simulink model "three_time_scale"  (R2015a)
settings: Solver=ode45  StartTime=0.0  StopTime=30000.0  RelTol=1e-3
values from neighbouring files (symbols this model uses):
  alpha = 0.25    [fast_nullcline_winged_cusp.m]    (also in relay_model_bistability.m; relay_model_bistability2.m)
  beta = 0.5    [fast_nullcline_winged_cusp.m]    (also in relay_model_bistability.m; relay_model_bistability2.m = 0.25)
  delta = 0.5    [fast_nullcline_winged_cusp.m]    (also in relay_model_bistability.m = 0.3; relay_model_bistability2.m = 0.3)
  gamma = 0.5    [fast_nullcline_winged_cusp.m]    (also in relay_model_bistability.m = 1; relay_model_bistability2.m = 1)
undefined symbols (not defined in the file or in its folder): xu
libraries: simulink x1
settings Model: CovModelRefEnable=off  Creator=rajiv  LastModifiedBy=rajiv
settings DataIOCC: SaveFormat=Dataset
settings HardwareCC: ProdBitPerPointer=64  ProdLargestAtomicFloat=Float  ProdIntDivRoundTo=Zero  ProdEndianess=LittleEndian  ProdHWDeviceType=Specified
settings GRTTargetCC: GeneratePreprocessorConditionals=Use local settings

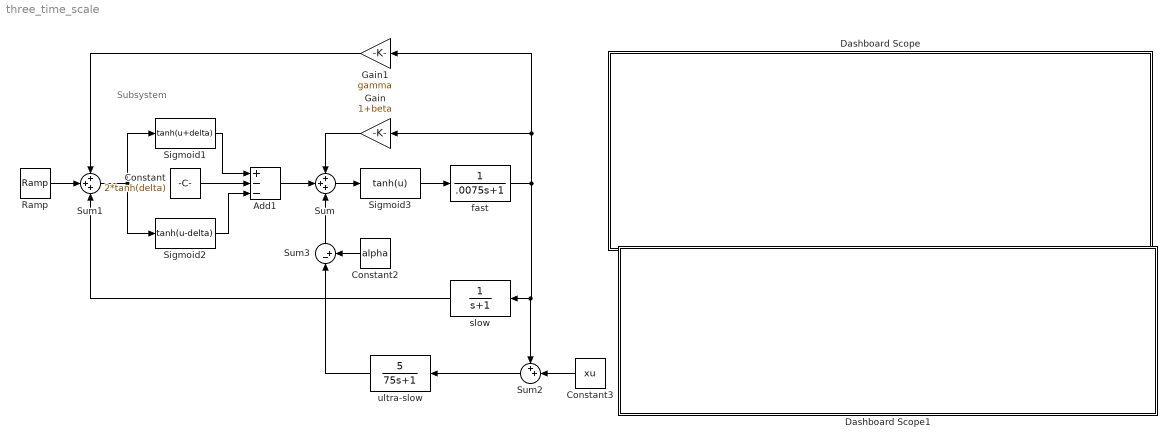
== system three_time_scale ==
  note: Subsystem
  Add1 : Sum  Inputs=+--
  Constant : Constant  Value=2*tanh(delta)
  Constant2 : Constant  Value=alpha
  Constant3 : Constant  Value=xu
  Dashboard Scope : Subsystem  DialogController=hmiCreateDDGDialog  IsWebBlock=on  mask(MWDashboardBlock){webBlockId=8879f959-95f0-45f4-b2bb-9dff7a2f39be, webBlockType=sdiscope, ShowInitialText=on, HMISrcModelName=three_time_scale}
      mask prompts: webBlockId "WebBlock Id"; webBlockType "WebBlock Type"; HMISrcModelName "Source Model"
      mask Help: helpview([docroot '/mapfiles/simulink.map'], 'hmi_scope')
      mask Display:
      | if strcmp(get_param(bdroot(gcb),'BlockDiagramType'), 'library')
      |     image([(matlabroot) '/toolbox/simulink/hmi/icons/DashboardScope.png']);
      | end
  Dashboard Scope1 : Subsystem  DialogController=hmiCreateDDGDialog  IsWebBlock=on  mask(MWDashboardBlock){webBlockId=d038109c-32c2-46cf-8e43-db6f4b827823, webBlockType=sdiscope, ShowInitialText=on, HMISrcModelName=three_time_scale}
      mask prompts: webBlockId "WebBlock Id"; webBlockType "WebBlock Type"; HMISrcModelName "Source Model"
      mask Help: helpview([docroot '/mapfiles/simulink.map'], 'hmi_scope')
      mask Display:
      | if strcmp(get_param(bdroot(gcb),'BlockDiagramType'), 'library')
      |     image([(matlabroot) '/toolbox/simulink/hmi/icons/DashboardScope.png']);
      | end
  Gain : Gain  Gain=1+beta
  Gain1 : Gain  Gain=gamma
  Ramp : simulink/Sources/Ramp  slope=6e-5  start=0  X0=0
  Sigmoid1 : Fcn  Expr=tanh(u+delta)
  Sigmoid2 : Fcn  Expr=tanh(u-delta)
  Sigmoid3 : Fcn  Expr=tanh(u)
  Sum : Sum  Inputs=+++
  Sum1 : Sum  Inputs=+++
  Sum2 : Sum  Inputs=++|
  Sum3 : Sum  Inputs=|-+
  fast : TransferFcn  Denominator=[.0075 1]
  slow : TransferFcn  Denominator=[1 1]
  ultra-slow : TransferFcn  Numerator=[5]  Denominator=[75 1]
  wires:
  Sum/1 -> Sigmoid3/1
  Constant/1 -> Add1/2
  Add1/1 -> Sum/2
  Sum1/1 -> Sigmoid2/1, Sigmoid1/1
  Sigmoid2/1 -> Add1/3
  Sigmoid1/1 -> Add1/1
  Gain/1 -> Sum/1
  slow/1 -> Sum1/3
  Gain1/1 -> Sum1/1
  Sigmoid3/1 -> fast/1
  fast/1 -> slow/1, Sum2/1, Gain1/1, Gain/1
  Sum3/1 -> Sum/3
  Constant2/1 -> Sum3/2
  ultra-slow/1 -> Sum3/1
  Sum2/1 -> ultra-slow/1
  Constant3/1 -> Sum2/2
  Ramp/1 -> Sum1/2

== system three_time_scale/Dashboard Scope ==

== system three_time_scale/Dashboard Scope1 ==
